simulink library "OutRspChkLib"  (R2018b)
settings: Solver=VariableStepAuto  StartTime=0.0  StopTime=10.0  RelTol=1e-3
undefined symbols (not defined in the file or in its folder): MdRspLocal2
settings Model: Creator=sn2xws  LastModifiedBy=sn2xws

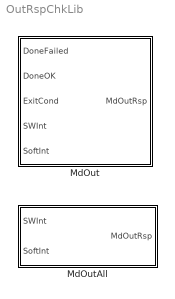
== system OutRspChkLib ==
  MdOut : Subsystem
  MdOutAll : Subsystem

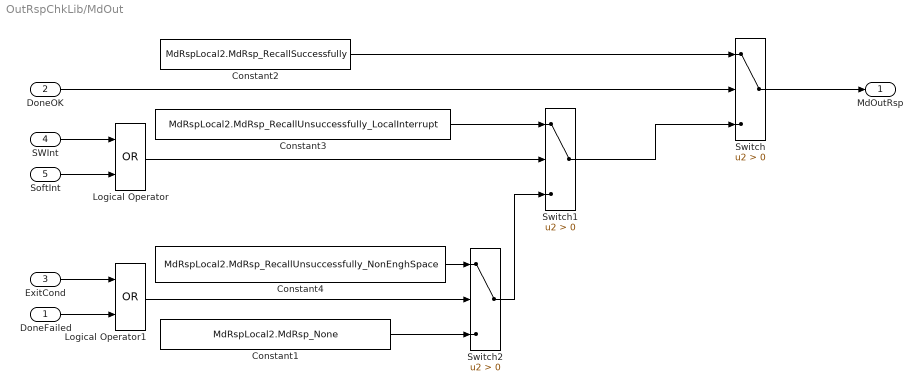
== system OutRspChkLib/MdOut ==
  DoneFailed : Inport
  DoneOK : Inport  Port=2
  ExitCond : Inport  Port=3
  SWInt : Inport  Port=4
  SoftInt : Inport  Port=5
  Constant1 : Constant  Value=MdRspLocal2.MdRsp_None  OutDataTypeStr=Enum:MdRspLocal2
  Constant2 : Constant  Value=MdRspLocal2.MdRsp_RecallSuccessfully  OutDataTypeStr=Enum:MdRspLocal2
  Constant3 : Constant  Value=MdRspLocal2.MdRsp_RecallUnsuccessfully_LocalInterrupt  OutDataTypeStr=Enum:MdRspLocal2
  Constant4 : Constant  Value=MdRspLocal2.MdRsp_RecallUnsuccessfully_NonEnghSpace  OutDataTypeStr=Enum:MdRspLocal2
  Logical Operator : Logic  Operator=OR  AllPortsSameDT=off  OutDataTypeStr=boolean
  Logical Operator1 : Logic  Operator=OR  AllPortsSameDT=off  OutDataTypeStr=boolean
  Switch : Switch  Criteria=u2 > Threshold
  Switch1 : Switch  Criteria=u2 > Threshold
  Switch2 : Switch  Criteria=u2 > Threshold
  MdOutRsp : Outport
  wires:
  ExitCond/1 -> Logical Operator1/1
  Switch/1 -> MdOutRsp/1
  DoneFailed/1 -> Logical Operator1/2
  Logical Operator1/1 -> Switch2/2
  Switch2/1 -> Switch1/3
  SWInt/1 -> Logical Operator/1
  SoftInt/1 -> Logical Operator/2
  Constant2/1 -> Switch/1
  Switch1/1 -> Switch/3
  Constant3/1 -> Switch1/1
  Logical Operator/1 -> Switch1/2
  Constant1/1 -> Switch2/3
  DoneOK/1 -> Switch/2
  Constant4/1 -> Switch2/1

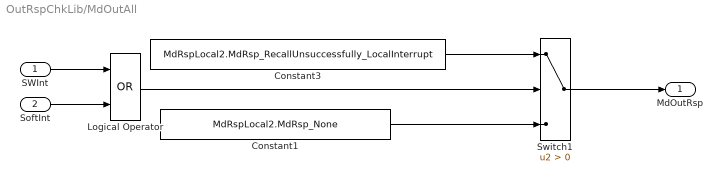
== system OutRspChkLib/MdOutAll ==
  SWInt : Inport
  SoftInt : Inport  Port=2
  Constant1 : Constant  Value=MdRspLocal2.MdRsp_None  OutDataTypeStr=Enum:MdRspLocal2
  Constant3 : Constant  Value=MdRspLocal2.MdRsp_RecallUnsuccessfully_LocalInterrupt  OutDataTypeStr=Enum:MdRspLocal2
  Logical Operator : Logic  Operator=OR  AllPortsSameDT=off  OutDataTypeStr=boolean
  Switch1 : Switch  Criteria=u2 > Threshold
  MdOutRsp : Outport
  wires:
  SWInt/1 -> Logical Operator/1
  Constant1/1 -> Switch1/3
  Constant3/1 -> Switch1/1
  Logical Operator/1 -> Switch1/2
  Switch1/1 -> MdOutRsp/1
  SoftInt/1 -> Logical Operator/2
